simulink model "MotorCooling"  (R2021a)
settings: Solver=FixedStepAuto  StartTime=0.0  StopTime=1373  FixedStep=1  RelTol=1e-3
values from neighbouring files (symbols this model uses):
  Cm = Motor_cooling_max_power/(Cp*(Tm-Tamb))    [Motor_Cooling.m]
  Cp = 4182    [Motor_Cooling.m]
  mCp = 1350    [Motor_Cooling.m]
  Mm = 23.69    [Motor_Cooling.m]
  Tamb = 18    [Motor_Cooling.m]
  Tmotor_i = 20    [Motor_Cooling.m]
settings Model: Creator=LENOVO  LastModifiedBy=LENOVO

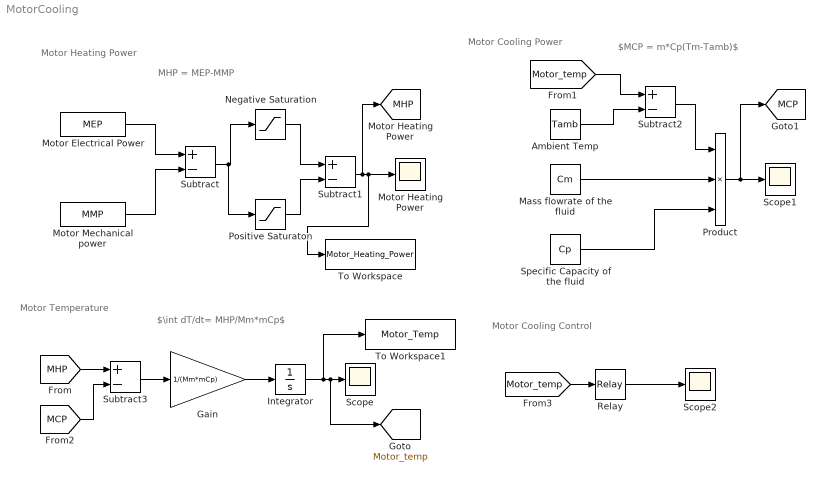
== system MotorCooling ==
  note: Motor Cooling Control
  note: $MCP = m*Cp(Tm-Tamb)$
  note: Motor Cooling Power
  note: $\int dT/dt= MHP/Mm*mCp$
  note: Motor Temperature
  note: Motor Heating Power
  note: MHP = MEP-MMP
  Ambient Temp : Constant  Value=Tamb
  Gain : Gain  Gain=1/(Mm*mCp)
  Integrator : Integrator  InitialCondition=Tmotor_i
  "Mass flowrate of the fluid " : Constant  Value=Cm
  Motor Electrical Power : FromWorkspace  VariableName=MEP
  Motor Mechanical power : FromWorkspace  VariableName=MMP
  Motor Heating Power : Scope
  Negative Saturation : Saturate  UpperLimit=inf  LowerLimit=0
  Positive Saturaton : Saturate  UpperLimit=0  LowerLimit=-inf
  Product : Product  Inputs=3
  Relay : Relay
  Scope : Scope
  Scope1 : Scope
  Scope2 : Scope
  Specific Capacity of the fluid : Constant  Value=Cp
  Subtract{,1..3} (4 alike) : Sum  Inputs=+-
  To Workspace : ToWorkspace  VariableName=Motor_Heating_Power  SaveFormat=Timeseries  SampleTime=-1
  To Workspace1 : ToWorkspace  VariableName=Motor_Temp  SaveFormat=Timeseries  SampleTime=-1
  tag scope: MCP=global, MHP=global, Motor_temp=global
  wires:
  Motor Electrical Power/1 -> Subtract/1
  Motor Mechanical power/1 -> Subtract/2
  Subtract/1 -> Positive Saturaton/1, Negative Saturation/1
  Negative Saturation/1 -> Subtract1/1
  Subtract1/1 -> Motor Heating Power/1, To Workspace/1, [MHP]
  Positive Saturaton/1 -> Subtract1/2
  Gain/1 -> Integrator/1
  Integrator/1 -> To Workspace1/1, [Motor_temp], Scope/1
  [Motor_temp] -> Subtract2/1
  Ambient Temp/1 -> Subtract2/2
  Subtract2/1 -> Product/1
  "Mass flowrate of the fluid "/1 -> Product/2
  Specific Capacity of the fluid/1 -> Product/3
  Product/1 -> [MCP], Scope1/1
  [MHP] -> Subtract3/1
  [MCP] -> Subtract3/2
  Subtract3/1 -> Gain/1
  [Motor_temp] -> Relay/1
  Relay/1 -> Scope2/1
